simulink library "checkVoltage"  (R2012b)
settings: Solver=ode45  StartTime=0.0  StopTime=10.0  RelTol=1e-3
libraries: dspstat3 x1
settings Model: Creator=huytbvo  LastModifiedBy=forrest

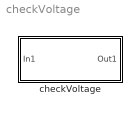
== system checkVoltage ==
  checkVoltage : Subsystem

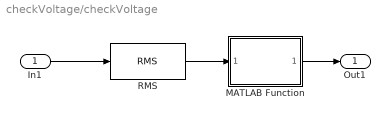
== system checkVoltage/checkVoltage ==
  In1 : Inport
  MATLAB Function : MATLAB Function  TreatAsAtomicUnit=on
  RMS : dspstat3/RMS  run=off  reset_popup=None  InputProcessing=Columns as channels (frame based)  directionMode=Each column  dimension=1  treatSBRowAsCol=on
  Out1 : Outport
  wires:
  In1/1 -> RMS/1
  RMS/1 -> MATLAB Function/1(rmsVoltage)
  MATLAB Function/1(isWorking) -> Out1/1

== matlab function checkVoltage/MATLAB Function ==
  data: rmsVoltage input; isWorking output



function isWorking = checkRmsVoltage(rmsVoltage)

isWorking = 0;
if(rmsVoltage >= 110 && rmsVoltage <=120)
    isWorking = 1;

end
